simulink model "controlo_atitude_sens_atuad_GulfVsim"  (R2020b)
settings: Solver=VariableStepAuto  StartTime=0.0  StopTime=100  RelTol=1e-3
values from neighbouring files (symbols this model uses):
  a = [ ... (first row only)    [espaco_estados_GulfV.m]
  aa0 = 7.17*deg    (= 0.125140107368)    [variaveis_GulfV.m]
  b = [ ... (first row only)    [espaco_estados_GulfV.m]
  F = inv(G)    [controlo_atitude_GulfV.m]
  k_lqr = lqr(a,b,q,r)    [controlo_atitude_GulfV.m]
  tt0 = gg0+aa0    (= 0.125140107368)    [variaveis_GulfV.m]
  u0 = 105.1*kn    (= 54.06344)    [variaveis_GulfV.m]
libraries: simulink x3
settings Model: Creator=Admin  LastModifiedBy=Admin

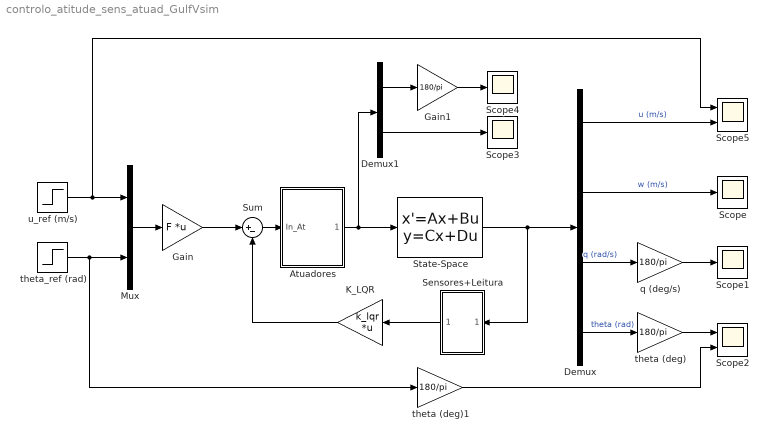
== system controlo_atitude_sens_atuad_GulfVsim ==
  Atuadores : Subsystem
  Demux : Demux
  Demux1 : Demux  Outputs=2
  Gain : Gain  Gain=F  Multiplication=Matrix(K*u)
  Gain1 : Gain  Gain=180/pi
  K_LQR : Gain  Gain=k_lqr  Multiplication=Matrix(K*u)
  Mux : Mux  Inputs=2
  Scope{,1,3..4} (4 alike) : Scope
  Scope2 : Scope  NumInputPorts=2
  Scope5 : Scope  NumInputPorts=2
  Sensores+Leitura : Subsystem
  State-Space : StateSpace  A=a  B=b  C=eye(4)  D=zeros(4,2)  InitialCondition=0
  Sum : Sum  Inputs=|+-
  q (deg/s) : Gain  Gain=180/pi
  theta (deg) : Gain  Gain=180/pi
  theta (deg)1 : Gain  Gain=180/pi
  theta_ref (rad) : Step  Time=5  After=0.0873  SampleTime=0
  u_ref (m/s) : Step  Time=50  After=2  SampleTime=0
  wires:
  Gain1/1 -> Scope4/1
  theta (deg)1/1 -> Scope2/2
  Demux1/2 -> Scope3/1
  u_ref (m/s)/1 -> Scope5/1, Mux/1
  Demux/1 -> Scope5/2  "u (m/s)"
  Demux/3 -> q (deg/s)/1  "q (rad/s)"
  q (deg/s)/1 -> Scope1/1
  Demux1/1 -> Gain1/1
  theta_ref (rad)/1 -> theta (deg)1/1, Mux/2
  theta (deg)/1 -> Scope2/1
  Demux/4 -> theta (deg)/1  "theta (rad)"
  K_LQR/1 -> Sum/2
  Demux/2 -> Scope/1  "w (m/s)"
  State-Space/1 -> Sensores+Leitura/1(In1), Demux/1
  Sensores+Leitura/1(Out2) -> K_LQR/1
  Gain/1 -> Sum/1
  Sum/1 -> Atuadores/1(In_At)
  Mux/1 -> Gain/1
  Atuadores/1(Out_At) -> Demux1/1, State-Space/1

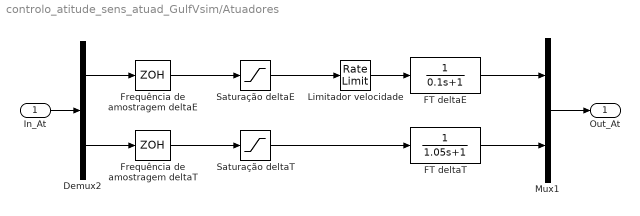
== system controlo_atitude_sens_atuad_GulfVsim/Atuadores ==
  In_At : Inport
  Demux2 : Demux  Outputs=2
  FT deltaE : TransferFcn  Denominator=[0.1 1]
  FT deltaT : TransferFcn  Denominator=[1.05 1]
  Frequência de amostragem deltaT : ZeroOrderHold  SampleTime=-1
  "Frequência de amostragem deltaE " : ZeroOrderHold  SampleTime=1/40
  Limitador velocidade : RateLimiter  SampleTimeMode=inherited
  Mux1 : Mux  Inputs=2
  Saturação deltaE : Saturate  UpperLimit=28*(pi/180)  LowerLimit=-21*(pi/180)
  Saturação deltaT : Saturate  UpperLimit=0.27  LowerLimit=-0.73
  Out_At : Outport
  wires:
  Demux2/2 -> Frequência de amostragem deltaT/1
  "Frequência de amostragem deltaE "/1 -> Saturação deltaE/1
  Demux2/1 -> "Frequência de amostragem deltaE "/1
  Mux1/1 -> Out_At/1
  FT deltaE/1 -> Mux1/1
  In_At/1 -> Demux2/1
  Saturação deltaE/1 -> Limitador velocidade/1
  Saturação deltaT/1 -> FT deltaT/1
  Limitador velocidade/1 -> FT deltaE/1
  Frequência de amostragem deltaT/1 -> Saturação deltaT/1
  FT deltaT/1 -> Mux1/2

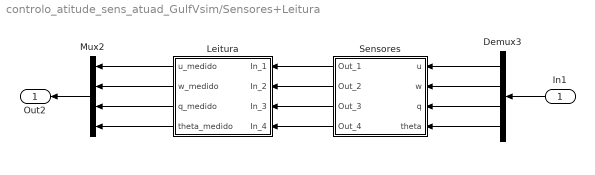
== system controlo_atitude_sens_atuad_GulfVsim/Sensores+Leitura ==
  In1 : Inport
  Demux3 : Demux
  Leitura : Subsystem
  Mux2 : Mux
  Sensores : Subsystem
  Out2 : Outport
  wires:
  Mux2/1 -> Out2/1
  In1/1 -> Demux3/1
  Leitura/1(u_medido) -> Mux2/1
  Leitura/2(w_medido) -> Mux2/2
  Leitura/3(q_medido) -> Mux2/3
  Leitura/4(theta_medido) -> Mux2/4
  Demux3/1 -> Sensores/1(u)
  Demux3/2 -> Sensores/2(w)
  Demux3/3 -> Sensores/3(q)
  Demux3/4 -> Sensores/4(theta)
  Sensores/1(Out_1) -> Leitura/1(In_1)
  Sensores/2(Out_2) -> Leitura/2(In_2)
  Sensores/3(Out_3) -> Leitura/3(In_3)
  Sensores/4(Out_4) -> Leitura/4(In_4)

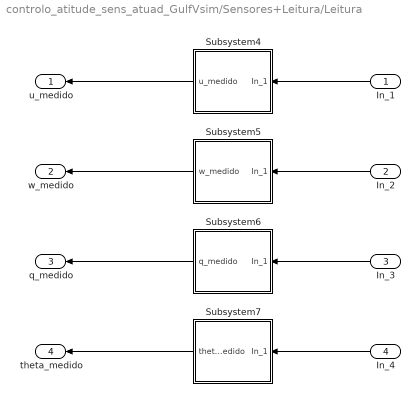
== system controlo_atitude_sens_atuad_GulfVsim/Sensores+Leitura/Leitura ==
  In_1 : Inport
  In_2 : Inport  Port=2
  In_3 : Inport  Port=3
  In_4 : Inport  Port=4
  Subsystem4 : Subsystem
  Subsystem5 : Subsystem
  Subsystem6 : Subsystem
  Subsystem7 : Subsystem
  u_medido : Outport
  w_medido : Outport  Port=2
  q_medido : Outport  Port=3
  theta_medido : Outport  Port=4
  wires:
  In_2/1 -> Subsystem5/1(In_1)
  In_4/1 -> Subsystem7/1(In_1)
  Subsystem7/1(theta_medido) -> theta_medido/1
  Subsystem6/1(q_medido) -> q_medido/1
  Subsystem5/1(w_medido) -> w_medido/1
  In_1/1 -> Subsystem4/1(In_1)
  Subsystem4/1(u_medido) -> u_medido/1
  In_3/1 -> Subsystem6/1(In_1)

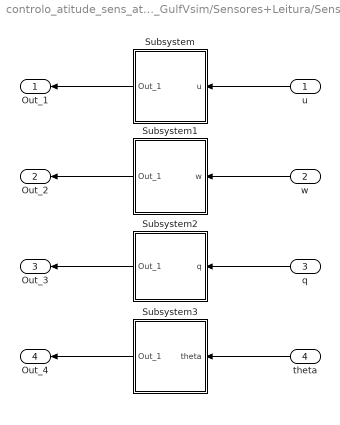
== system controlo_atitude_sens_atuad_GulfVsim/Sensores+Leitura/Sensores ==
  u : Inport
  w : Inport  Port=2
  q : Inport  Port=3
  theta : Inport  Port=4
  Subsystem : Subsystem
  Subsystem1 : Subsystem
  Subsystem2 : Subsystem
  Subsystem3 : Subsystem
  Out_1 : Outport
  Out_2 : Outport  Port=2
  Out_3 : Outport  Port=3
  Out_4 : Outport  Port=4
  wires:
  Subsystem2/1(Out_1) -> Out_3/1
  q/1 -> Subsystem2/1(q)
  theta/1 -> Subsystem3/1(theta)
  Subsystem3/1(Out_1) -> Out_4/1
  u/1 -> Subsystem/1(u)
  w/1 -> Subsystem1/1(w)
  Subsystem/1(Out_1) -> Out_1/1
  Subsystem1/1(Out_1) -> Out_2/1

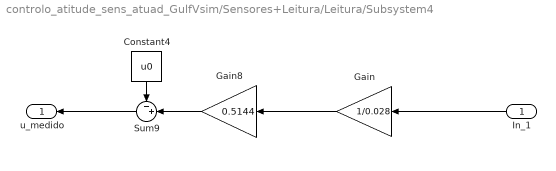
== system controlo_atitude_sens_atuad_GulfVsim/Sensores+Leitura/Leitura/Subsystem4 ==
  In_1 : Inport
  Constant4 : Constant  Value=u0
  Gain : Gain  Gain=1/0.028
  Gain8 : Gain  Gain=0.5144
  Sum9 : Sum  Inputs=-+|
  u_medido : Outport
  wires:
  Constant4/1 -> Sum9/1
  In_1/1 -> Gain/1
  Gain8/1 -> Sum9/2
  Gain/1 -> Gain8/1
  Sum9/1 -> u_medido/1

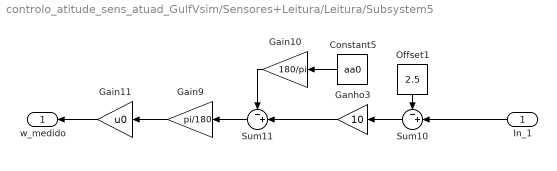
== system controlo_atitude_sens_atuad_GulfVsim/Sensores+Leitura/Leitura/Subsystem5 ==
  In_1 : Inport
  Constant5 : Constant  Value=aa0
  Gain10 : Gain  Gain=180/pi
  Gain11 : Gain  Gain=u0
  Gain9 : Gain  Gain=pi/180
  Ganho3 : Gain  Gain=10
  Offset1 : Constant  Value=2.5
  Sum10 : Sum  Inputs=-+|
  Sum11 : Sum  Inputs=-+|
  w_medido : Outport
  wires:
  Sum11/1 -> Gain9/1
  Constant5/1 -> Gain10/1
  Ganho3/1 -> Sum11/2
  In_1/1 -> Sum10/2
  Gain11/1 -> w_medido/1
  Gain9/1 -> Gain11/1
  Gain10/1 -> Sum11/1
  Offset1/1 -> Sum10/1
  Sum10/1 -> Ganho3/1

== system controlo_atitude_sens_atuad_GulfVsim/Sensores+Leitura/Leitura/Subsystem6 ==
  In_1 : Inport
  Gain12 : Gain  Gain=pi/180
  Ganho4 : Gain  Gain=1/0.06
  q_medido : Outport
  wires:
  Ganho4/1 -> Gain12/1
  In_1/1 -> Ganho4/1
  Gain12/1 -> q_medido/1

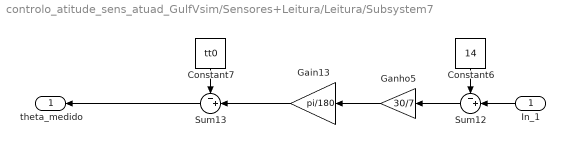
== system controlo_atitude_sens_atuad_GulfVsim/Sensores+Leitura/Leitura/Subsystem7 ==
  In_1 : Inport
  Constant6 : Constant  Value=14
  Constant7 : Constant  Value=tt0
  Gain13 : Gain  Gain=pi/180
  Ganho5 : Gain  Gain=30/7
  Sum12 : Sum  Inputs=-+|
  Sum13 : Sum  Inputs=-+|
  theta_medido : Outport
  wires:
  Constant7/1 -> Sum13/1
  Sum12/1 -> Ganho5/1
  Sum13/1 -> theta_medido/1
  Gain13/1 -> Sum13/2
  Ganho5/1 -> Gain13/1
  Constant6/1 -> Sum12/1
  In_1/1 -> Sum12/2

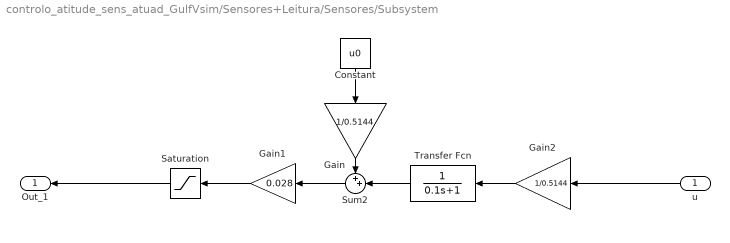
== system controlo_atitude_sens_atuad_GulfVsim/Sensores+Leitura/Sensores/Subsystem ==
  u : Inport
  Constant : Constant  Value=u0
  Gain : Gain  Gain=1/0.5144
  Gain1 : Gain  Gain=0.028
  Gain2 : Gain  Gain=1/0.5144
  Saturation : Saturate  UpperLimit=28  LowerLimit=0
  Sum2 : Sum  Inputs=++|
  Transfer Fcn : TransferFcn  Denominator=[0.1 1]
  Out_1 : Outport
  wires:
  Sum2/1 -> Gain1/1
  Saturation/1 -> Out_1/1
  Gain1/1 -> Saturation/1
  u/1 -> Gain2/1
  Transfer Fcn/1 -> Sum2/2
  Constant/1 -> Gain/1
  Gain2/1 -> Transfer Fcn/1
  Gain/1 -> Sum2/1

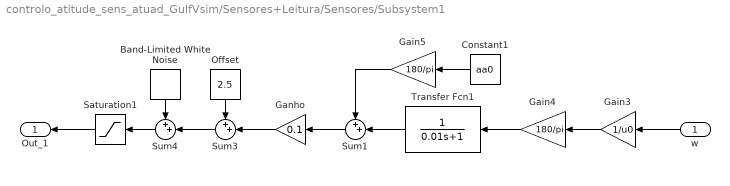
== system controlo_atitude_sens_atuad_GulfVsim/Sensores+Leitura/Sensores/Subsystem1 ==
  w : Inport
  Band-Limited White Noise : simulink/Sources/Band-Limited White Noise  Cov=[(0.005)^2/40]  Ts=1/40  seed=[23341]
  Constant1 : Constant  Value=aa0
  Gain3 : Gain  Gain=1/u0
  Gain4 : Gain  Gain=180/pi
  Gain5 : Gain  Gain=180/pi
  Ganho : Gain  Gain=0.1
  Offset : Constant  Value=2.5
  Saturation1 : Saturate  UpperLimit=5  LowerLimit=0
  Sum1 : Sum  Inputs=++|
  Sum3 : Sum  Inputs=++|
  Sum4 : Sum  Inputs=++|
  Transfer Fcn1 : TransferFcn  Denominator=[0.01 1]
  Out_1 : Outport
  wires:
  Gain5/1 -> Sum1/1
  Sum1/1 -> Ganho/1
  Offset/1 -> Sum3/1
  Constant1/1 -> Gain5/1
  Ganho/1 -> Sum3/2
  Gain4/1 -> Transfer Fcn1/1
  Sum4/1 -> Saturation1/1
  Band-Limited White Noise/1 -> Sum4/1
  Gain3/1 -> Gain4/1
  Transfer Fcn1/1 -> Sum1/2
  Sum3/1 -> Sum4/2
  w/1 -> Gain3/1
  Saturation1/1 -> Out_1/1

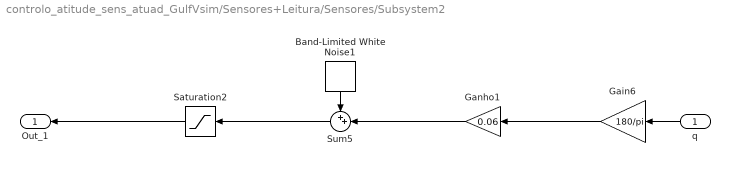
== system controlo_atitude_sens_atuad_GulfVsim/Sensores+Leitura/Sensores/Subsystem2 ==
  q : Inport
  Band-Limited White Noise1 : simulink/Sources/Band-Limited White Noise  Cov=[(0.002)^2/40]  Ts=1/40  seed=[23341]
  Gain6 : Gain  Gain=180/pi
  Ganho1 : Gain  Gain=0.06
  Saturation2 : Saturate  UpperLimit=3  LowerLimit=-3
  Sum5 : Sum  Inputs=++|
  Out_1 : Outport
  wires:
  Sum5/1 -> Saturation2/1
  Ganho1/1 -> Sum5/2
  Band-Limited White Noise1/1 -> Sum5/1
  q/1 -> Gain6/1
  Saturation2/1 -> Out_1/1
  Gain6/1 -> Ganho1/1

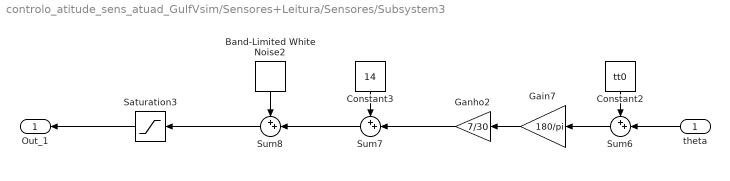
== system controlo_atitude_sens_atuad_GulfVsim/Sensores+Leitura/Sensores/Subsystem3 ==
  theta : Inport
  Band-Limited White Noise2 : simulink/Sources/Band-Limited White Noise  Cov=[(0.25)^2/40]  Ts=1/40  seed=[23341]
  Constant2 : Constant  Value=tt0
  Constant3 : Constant  Value=14
  Gain7 : Gain  Gain=180/pi
  Ganho2 : Gain  Gain=7/30
  Saturation3 : Saturate  UpperLimit=28  LowerLimit=0
  Sum6 : Sum  Inputs=++|
  Sum7 : Sum  Inputs=++|
  Sum8 : Sum  Inputs=++|
  Out_1 : Outport
  wires:
  Sum7/1 -> Sum8/2
  Gain7/1 -> Ganho2/1
  Constant2/1 -> Sum6/1
  Constant3/1 -> Sum7/1
  Sum8/1 -> Saturation3/1
  Ganho2/1 -> Sum7/2
  Sum6/1 -> Gain7/1
  Saturation3/1 -> Out_1/1
  Band-Limited White Noise2/1 -> Sum8/1
  theta/1 -> Sum6/2
